simulink model "LateralControllerLQR"  (R2022a)
settings: Solver=FixedStepAuto  StartTime=0.0  StopTime=10.0  RelTol=1e-3
undefined symbols (not defined in the file): LateralControllers_FeedbackGainLQR
libraries: CarMaker4SL x8
settings Model: Creator=krisz  LastModifiedBy=Krisztian

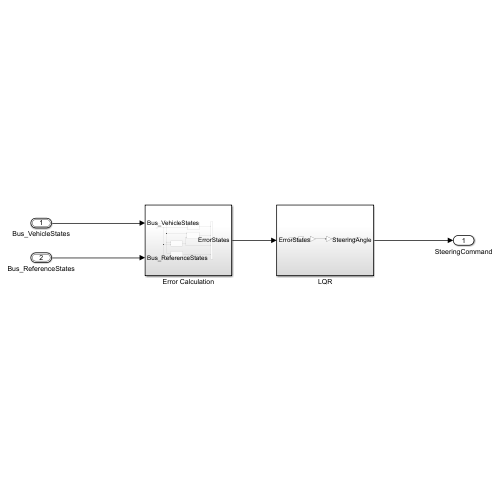
[thumbnail: Simulink's stored preview of the top-level diagram]
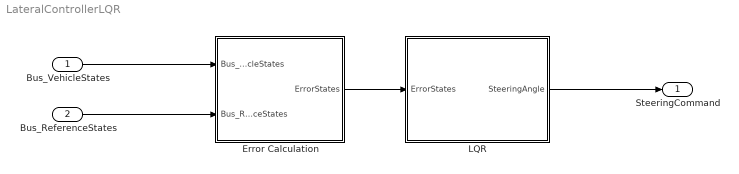
== system LateralControllerLQR ==
  Bus_VehicleStates : Inport  OutDataTypeStr=Bus: bus_VehicleStates
  Bus_ReferenceStates : Inport  Port=2  OutDataTypeStr=Bus: bus_ReferenceStates
  Error Calculation : Subsystem
  "LQR " : Subsystem
  SteeringCommand : Outport
  wires:
  Error Calculation/1(ErrorStates) -> "LQR "/1(ErrorStates)
  "LQR "/1(SteeringAngle) -> SteeringCommand/1
  Bus_ReferenceStates/1 -> Error Calculation/2(Bus_ReferenceStates)
  Bus_VehicleStates/1 -> Error Calculation/1(Bus_VehicleStates)

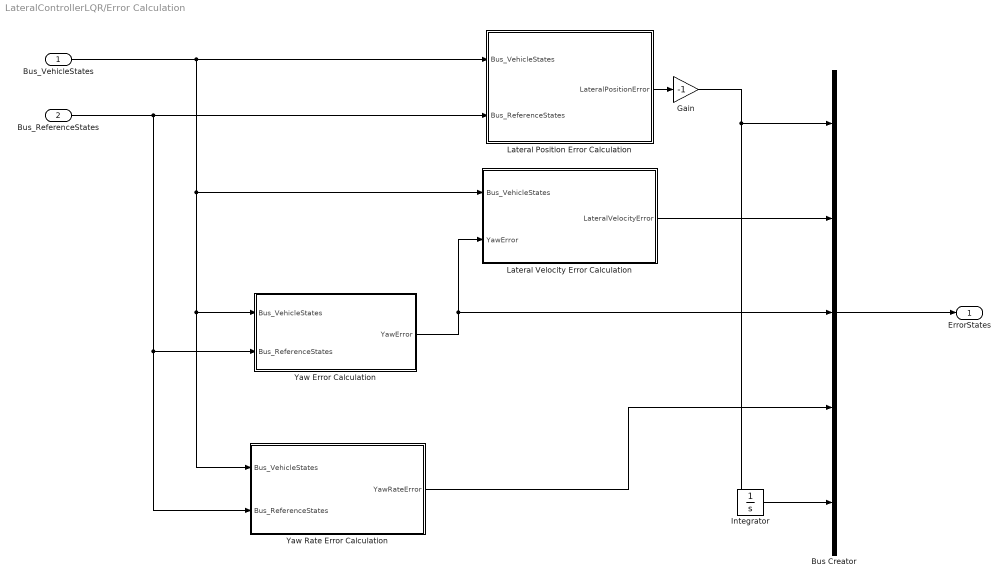
== system LateralControllerLQR/Error Calculation ==
  Bus_VehicleStates : Inport
  Bus_ReferenceStates : Inport  Port=2
  Bus Creator : BusCreator  Inputs=5  OutDataTypeStr=Bus: bus_ErrorStates
      settings: InheritFromInputs=off
  Gain : Gain  Gain=-1
  Integrator : Integrator
  Lateral Position Error Calculation : Subsystem
  Lateral Velocity Error Calculation : Subsystem
  Yaw Error Calculation : Subsystem
  Yaw Rate Error Calculation : Subsystem
  ErrorStates : Outport  OutDataTypeStr=Bus: bus_ErrorStates
  wires:
  Bus_VehicleStates/1 -> Lateral Position Error Calculation/1(Bus_VehicleStates), Yaw Rate Error Calculation/1(Bus_VehicleStates), Yaw Error Calculation/1(Bus_VehicleStates), Lateral Velocity Error Calculation/1(Bus_VehicleStates)
  Bus_ReferenceStates/1 -> Yaw Error Calculation/2(Bus_ReferenceStates), Yaw Rate Error Calculation/2(Bus_ReferenceStates), Lateral Position Error Calculation/2(Bus_ReferenceStates)
  Bus Creator/1 -> ErrorStates/1
  Yaw Rate Error Calculation/1(YawRateError) -> Bus Creator/4
  Yaw Error Calculation/1(YawError) -> Bus Creator/3, Lateral Velocity Error Calculation/2(YawError)
  Lateral Velocity Error Calculation/1(LateralVelocityError) -> Bus Creator/2
  Integrator/1 -> Bus Creator/5
  Lateral Position Error Calculation/1(LateralPositionError) -> Gain/1
  Gain/1 -> Integrator/1, Bus Creator/1

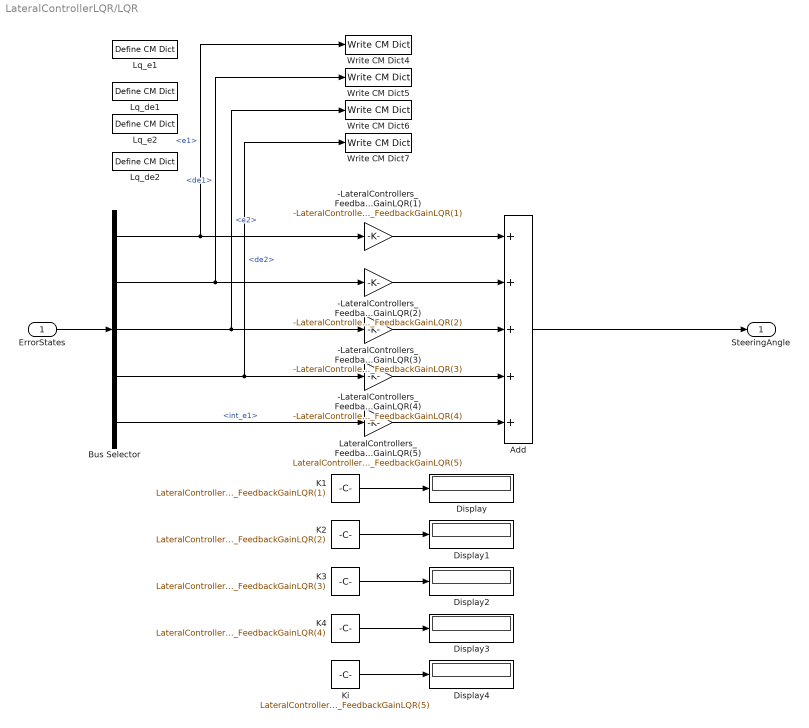
== system LateralControllerLQR/LQR  ==
  ErrorStates : Inport  OutDataTypeStr=Bus: bus_ErrorStates
  -LateralControllers_FeedbackGainLQR(1) : Gain  Gain=-LateralControllers_FeedbackGainLQR(1)
  -LateralControllers_FeedbackGainLQR(2) : Gain  Gain=-LateralControllers_FeedbackGainLQR(2)
  -LateralControllers_FeedbackGainLQR(3) : Gain  Gain=-LateralControllers_FeedbackGainLQR(3)
  -LateralControllers_FeedbackGainLQR(4) : Gain  Gain=-LateralControllers_FeedbackGainLQR(4)
  Add : Sum  Inputs=+++++
  Bus Selector : BusSelector  OutputSignals=e1,de1,e2,de2,int_e1
  Display{,1..4} (5 alike) : Display
  K1 : Constant  Value=LateralControllers_FeedbackGainLQR(1)
  K2 : Constant  Value=LateralControllers_FeedbackGainLQR(2)
  K3 : Constant  Value=LateralControllers_FeedbackGainLQR(3)
  K4 : Constant  Value=LateralControllers_FeedbackGainLQR(4)
  Ki : Constant  Value=LateralControllers_FeedbackGainLQR(5)
  LateralControllers_FeedbackGainLQR(5) : Gain  Gain=LateralControllers_FeedbackGainLQR(5)
  Lq_de1 : CarMaker4SL/Define CM Dict  xname=LQ_de1  xmono=off  xtype=Double4  xdvaplace=None  xnstates=0  xfirststate=0  xinitial=0
  Lq_de2 : CarMaker4SL/Define CM Dict  xname=LQ_de2  xmono=off  xtype=Double4  xdvaplace=None  xnstates=0  xfirststate=0  xinitial=0
  Lq_e1 : CarMaker4SL/Define CM Dict  xname=LQ_e1  xmono=off  xtype=Double4  xdvaplace=None  xnstates=0  xfirststate=0  xinitial=0
  Lq_e2 : CarMaker4SL/Define CM Dict  xname=LQ_e2  xmono=off  xtype=Double4  xdvaplace=None  xnstates=0  xfirststate=0  xinitial=0
  Write CM Dict4 : CarMaker4SL/Write CM Dict  xname=LQ_e1  xsync=off
  Write CM Dict5 : CarMaker4SL/Write CM Dict  xname=LQ_de1  xsync=off
  Write CM Dict6 : CarMaker4SL/Write CM Dict  xname=LQ_e2  xsync=off
  Write CM Dict7 : CarMaker4SL/Write CM Dict  xname=LQ_de2  xsync=off
  SteeringAngle : Outport
  wires:
  ErrorStates/1 -> Bus Selector/1
  Add/1 -> SteeringAngle/1
  LateralControllers_FeedbackGainLQR(5)/1 -> Add/5
  -LateralControllers_FeedbackGainLQR(4)/1 -> Add/4
  -LateralControllers_FeedbackGainLQR(3)/1 -> Add/3
  -LateralControllers_FeedbackGainLQR(2)/1 -> Add/2
  -LateralControllers_FeedbackGainLQR(1)/1 -> Add/1
  Bus Selector/5 -> LateralControllers_FeedbackGainLQR(5)/1  "<int_e1>"
  K1/1 -> Display/1
  K2/1 -> Display1/1
  K3/1 -> Display2/1
  K4/1 -> Display3/1
  Ki/1 -> Display4/1
  Bus Selector/2 -> Write CM Dict5/1, -LateralControllers_FeedbackGainLQR(2)/1  "<de1>"
  Bus Selector/3 -> Write CM Dict6/1, -LateralControllers_FeedbackGainLQR(3)/1  "<e2>"
  Bus Selector/4 -> Write CM Dict7/1, -LateralControllers_FeedbackGainLQR(4)/1  "<de2>"
  Bus Selector/1 -> Write CM Dict4/1, -LateralControllers_FeedbackGainLQR(1)/1  "<e1>"

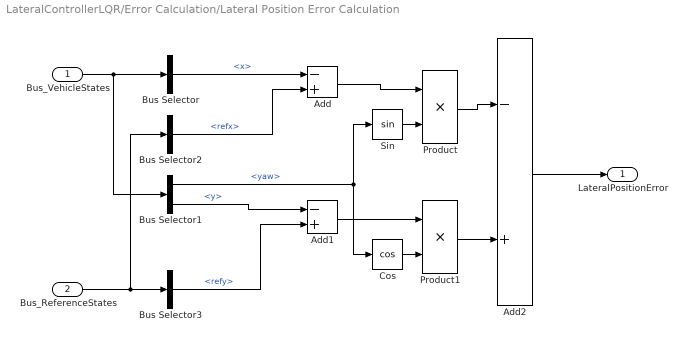
== system LateralControllerLQR/Error Calculation/Lateral Position Error Calculation ==
  Bus_VehicleStates : Inport  OutDataTypeStr=Bus: bus_VehicleStates
  Bus_ReferenceStates : Inport  Port=2  OutDataTypeStr=Bus: bus_ReferenceStates
  Add : Sum  Inputs=-+
  Add1 : Sum  Inputs=-+
  Add2 : Sum  Inputs=-+
  Bus Selector : BusSelector  OutputSignals=x
  Bus Selector1 : BusSelector  OutputSignals=yaw,y
  Bus Selector2 : BusSelector  OutputSignals=refx
  Bus Selector3 : BusSelector  OutputSignals=refy
  Cos : Trigonometry  Operator=cos
  Product : Product  Inputs=**
  Product1 : Product  Inputs=**
  Sin : Trigonometry
  LateralPositionError : Outport
  wires:
  Add2/1 -> LateralPositionError/1
  Product/1 -> Add2/1
  Product1/1 -> Add2/2
  Sin/1 -> Product/2
  Cos/1 -> Product1/2
  Add1/1 -> Product1/1
  Add/1 -> Product/1
  Bus_VehicleStates/1 -> Bus Selector1/1, Bus Selector/1
  Bus Selector/1 -> Add/1  "<x>"
  Bus Selector1/2 -> Add1/1  "<y>"
  Bus_ReferenceStates/1 -> Bus Selector2/1, Bus Selector3/1
  Bus Selector2/1 -> Add/2  "<refx>"
  Bus Selector3/1 -> Add1/2  "<refy>"
  Bus Selector1/1 -> Sin/1, Cos/1  "<yaw>"

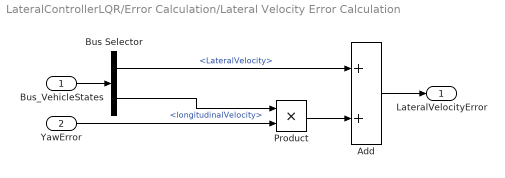
== system LateralControllerLQR/Error Calculation/Lateral Velocity Error Calculation ==
  Bus_VehicleStates : Inport  OutDataTypeStr=Bus: bus_VehicleStates
  YawError : Inport  Port=2
  Add : Sum
  Bus Selector : BusSelector  OutputSignals=LateralVelocity,longitudinalVelocity
  Product : Product  Inputs=**
  LateralVelocityError : Outport
  wires:
  Bus_VehicleStates/1 -> Bus Selector/1
  YawError/1 -> Product/2
  Bus Selector/2 -> Product/1  "<longitudinalVelocity>"
  Bus Selector/1 -> Add/1  "<LateralVelocity>"
  Product/1 -> Add/2
  Add/1 -> LateralVelocityError/1

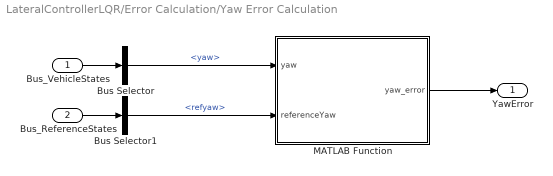
== system LateralControllerLQR/Error Calculation/Yaw Error Calculation ==
  Bus_VehicleStates : Inport  OutDataTypeStr=Bus: bus_VehicleStates
  Bus_ReferenceStates : Inport  Port=2  OutDataTypeStr=Bus: bus_ReferenceStates
  Bus Selector : BusSelector  OutputSignals=yaw
  Bus Selector1 : BusSelector  OutputSignals=refyaw
  MATLAB Function : MATLAB Function  TreatAsAtomicUnit=on
  YawError : Outport
  wires:
  Bus_VehicleStates/1 -> Bus Selector/1
  Bus_ReferenceStates/1 -> Bus Selector1/1
  Bus Selector/1 -> MATLAB Function/1(yaw)  "<yaw>"
  Bus Selector1/1 -> MATLAB Function/2(referenceYaw)  "<refyaw>"
  MATLAB Function/1(yaw_error) -> YawError/1

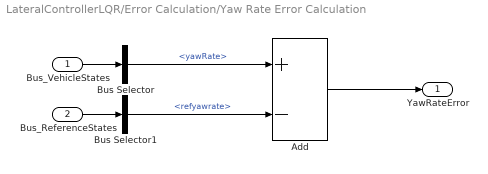
== system LateralControllerLQR/Error Calculation/Yaw Rate Error Calculation ==
  Bus_VehicleStates : Inport  OutDataTypeStr=Bus: bus_VehicleStates
  Bus_ReferenceStates : Inport  Port=2  OutDataTypeStr=Bus: bus_ReferenceStates
  Add : Sum  Inputs=+-
  Bus Selector : BusSelector  OutputSignals=yawRate
  Bus Selector1 : BusSelector  OutputSignals=refyawrate
  YawRateError : Outport
  wires:
  Bus_VehicleStates/1 -> Bus Selector/1
  Bus_ReferenceStates/1 -> Bus Selector1/1
  Bus Selector/1 -> Add/1  "<yawRate>"
  Add/1 -> YawRateError/1
  Bus Selector1/1 -> Add/2  "<refyawrate>"

== matlab function LateralControllerLQR/Error Calculation/Yaw Error Calculation/MATLAB Function ==
  data: yaw input; yaw_error output; referenceYaw input
function yaw_error = angle_diff(yaw, referenceYaw)
%#codegen
% yaw, referenceYaw: [rad]
% ePsi: heading error in [-pi, pi]

yaw_error = yaw - referenceYaw;  % = wrapToPi(yaw - referenceYaw)
end
